simulink model "calculate_mppt"  (R2018b)
settings: Solver=FixedStepDiscrete  StartTime=0.0  StopTime=10.0  RelTol=1e-3
settings Model: Creator=matlab  LastModifiedBy=matlab
settings DataIOCC: SaveOutput=off  SignalLogging=off  SaveTime=off
settings OptimizationCC: DefaultParameterBehavior=Inlined  EnhancedBackFolding=on  PassReuseOutputArgsAs=Individual arguments  OptimizeBlockOrder=speed  DifferentSizesBufferReuse=on  OptimizationCustomize=off
settings DebuggingCC: ParameterTunabilityLossMsg=error
settings SFSimCC: MATLABDynamicMemAlloc=off
settings RTWCC: SystemTargetFile=ert.tlc  TemplateMakefile=ert_default_tmf  PostCodeGenCommand=packNGo(buildInfo);  GenerateReport=on  IncludeHyperlinkInReport=on  LaunchReport=on  GenerateTraceInfo=on  GenerateTraceReport=on  GenerateTraceReportSl=on  GenerateTraceReportSf=on  GenerateTraceReportEml=on
settings CodeAppCC: ForceParamTrailComments=on  IgnoreCustomStorageClasses=off  OperatorAnnotations=on  SimulinkDataObjDesc=on  SFDataObjDesc=on  InsertBlockDesc=on
settings ERTTargetCC: TargetLangStandard=C99 (ISO)  GenerateSampleERTMain=on  InlinedParameterPlacement=NonHierarchical  ERTCustomFileTemplate=example_file_process.tlc

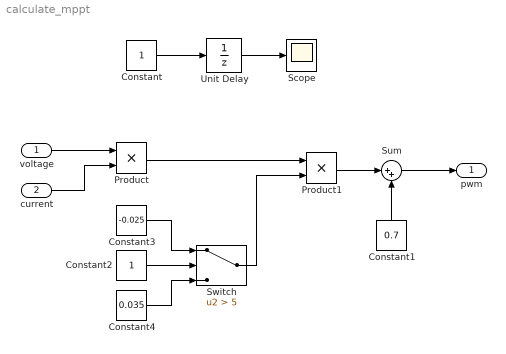
== system calculate_mppt ==
  voltage : Inport  OutDataTypeStr=AuroraVoltage  BusOutputAsStruct=on
  current : Inport  Port=2  OutDataTypeStr=AuroraCurrent  BusOutputAsStruct=on
  Constant : Constant
  Constant1 : Constant  Value=0.7
  Constant2 : Constant
  Constant3 : Constant  Value=-0.025
  Constant4 : Constant  Value=0.035
  Product : Product
  Product1 : Product
  Scope : Scope
  Sum : Sum  Inputs=|++
  Switch : Switch  Criteria=u2 > Threshold  Threshold=5
  Unit Delay : UnitDelay  SampleTime=-1
  pwm : Outport  OutDataTypeStr=AuroraPWM
  wires:
  Constant/1 -> Unit Delay/1
  Unit Delay/1 -> Scope/1
  Constant1/1 -> Sum/2
  Product/1 -> Product1/1
  Switch/1 -> Product1/2
  Product1/1 -> Sum/1
  Constant2/1 -> Switch/2
  Constant4/1 -> Switch/3
  Constant3/1 -> Switch/1
  voltage/1 -> Product/1
  current/1 -> Product/2
  Sum/1 -> pwm/1
